simulink model "merge2"  (R2022a)
settings: Solver=VariableStepAuto  StartTime=0.0  StopTime=10000.0  RelTol=1e-3
settings Model: Creator=kasturkoul  LastModifiedBy=kasturkoul

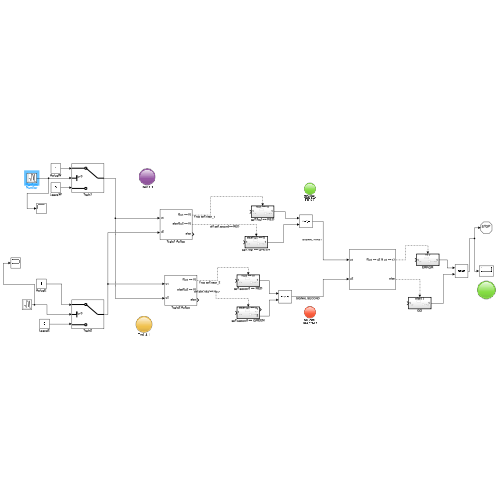
[thumbnail: Simulink's stored preview of the top-level diagram]
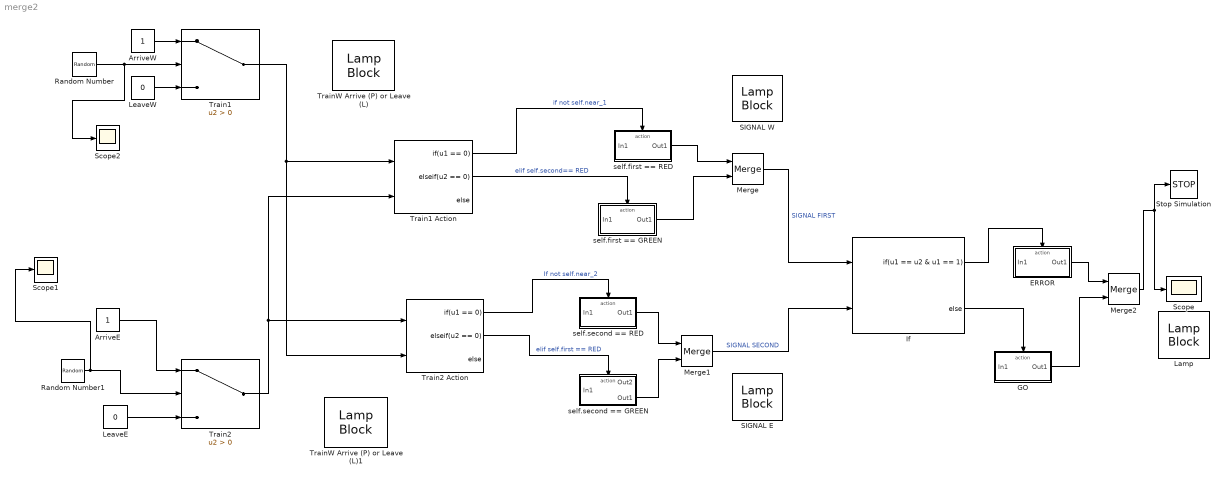
== system merge2 ==
  ArriveE : Constant
  ArriveW : Constant
  ERROR : Subsystem  TreatAsAtomicUnit=on
  GO : Subsystem  TreatAsAtomicUnit=on
  If : If  NumInputs=2  IfExpression=u1 == u2 & u1 == 1
  Lamp : LampBlock  LabelPosition=Hide
  LeaveE : Constant  Value=0
  LeaveW : Constant  Value=0
  Merge : Merge
  Merge1 : Merge
  Merge2 : Merge
  Random Number : RandomNumber  Variance=2  Seed=1  SampleTime=1
  Random Number1 : RandomNumber  SampleTime=0.1
  SIGNAL E : LampBlock  LabelPosition=Bottom
  SIGNAL W : LampBlock  LabelPosition=Bottom
  Scope : Scope
  Scope1 : Scope
  Scope2 : Scope
  Stop Simulation : Stop
  Train1 : Switch  Criteria=u2 > Threshold  SaturateOnIntegerOverflow=off  InputSameDT=off
  Train1 Action : If  NumInputs=2  IfExpression=u1 == 0  ElseIfExpressions=u2 == 0
  Train2 : Switch  Criteria=u2 > Threshold  SaturateOnIntegerOverflow=off  InputSameDT=off
  Train2 Action : If  NumInputs=2  IfExpression=u1 == 0  ElseIfExpressions=u2 == 0
  TrainW Arrive (P) or Leave (L) : LampBlock  LabelPosition=Bottom
  TrainW Arrive (P) or Leave (L)1 : LampBlock  LabelPosition=Bottom
  self.first == GREEN : Subsystem  TreatAsAtomicUnit=on
  self.first == RED : Subsystem  TreatAsAtomicUnit=on
  self.second == GREEN : Subsystem  TreatAsAtomicUnit=on
  self.second == RED : Subsystem  TreatAsAtomicUnit=on
  wires:
  self.second == GREEN/2(Out1) -> Merge1/2
  Random Number/1 -> Scope2/1, Train1/2
  Merge/1 -> If/1  "SIGNAL FIRST"
  Merge2/1 -> Scope/1, Stop Simulation/1
  LeaveW/1 -> Train1/3
  GO/1(Out1) -> Merge2/2
  self.second == RED/1(Out1) -> Merge1/1
  Train2 Action/2 -> self.second == GREEN/Action  "elif self.first == RED"
  If/2 -> GO/Action
  ArriveW/1 -> Train1/1
  Merge1/1 -> If/2  "SIGNAL SECOND"
  Random Number1/1 -> Scope1/1, Train2/2
  self.first == RED/1(Out1) -> Merge/1
  If/1 -> ERROR/Action
  Train1/1 -> Train2 Action/2, Train1 Action/1
  self.first == GREEN/1(Out1) -> Merge/2
  Train1 Action/2 -> self.first == GREEN/Action  "elif self.second== RED"
  Train2 Action/1 -> self.second == RED/Action  "If not self.near_2"
  ERROR/1(Out1) -> Merge2/1
  Train1 Action/1 -> self.first == RED/Action  "if not self.near_1"
  Train2/1 -> Train1 Action/2, Train2 Action/1
  LeaveE/1 -> Train2/3
  ArriveE/1 -> Train2/1

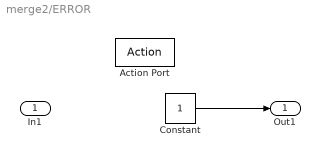
== system merge2/ERROR ==
  In1 : Inport
  Action Port : ActionPort  ActionPortLabel=if(u1 == u2 & u1 == 1)
  Constant : Constant
  Out1 : Outport
  wires:
  Constant/1 -> Out1/1

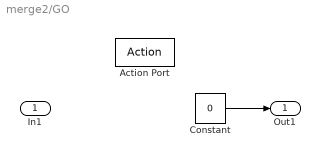
== system merge2/GO ==
  In1 : Inport
  Action Port : ActionPort  ActionPortLabel=else
  Constant : Constant  Value=0
  Out1 : Outport
  wires:
  Constant/1 -> Out1/1

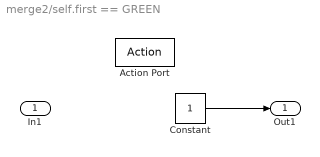
== system merge2/self.first == GREEN ==
  In1 : Inport
  Action Port : ActionPort  ActionPortLabel=elseif(u2 == 0)
  Constant : Constant
  Out1 : Outport
  wires:
  Constant/1 -> Out1/1

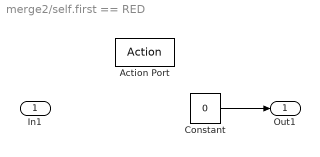
== system merge2/self.first == RED ==
  In1 : Inport
  Action Port : ActionPort  ActionPortLabel=if(u1 == 0)
  Constant : Constant  Value=0
  Out1 : Outport
  wires:
  Constant/1 -> Out1/1

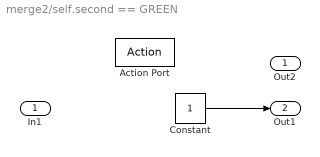
== system merge2/self.second == GREEN ==
  In1 : Inport
  Action Port : ActionPort  ActionPortLabel=elseif(u2 == 0)
  Constant : Constant
  Out2 : Outport
  Out1 : Outport  Port=2
  wires:
  Constant/1 -> Out1/1

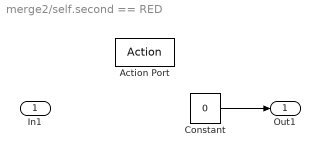
== system merge2/self.second == RED ==
  In1 : Inport
  Action Port : ActionPort  ActionPortLabel=if(u1 == 0)
  Constant : Constant  Value=0
  Out1 : Outport
  wires:
  Constant/1 -> Out1/1
